simulink model "dcmotor"  (R2020b)
settings: Solver=VariableStepAuto  StartTime=0.0  StopTime=10.0  RelTol=1e-3
settings Model: Creator=Aftab  LastModifiedBy=Aftab
settings DebuggingCC: SFMachineParentedDataDiag=error

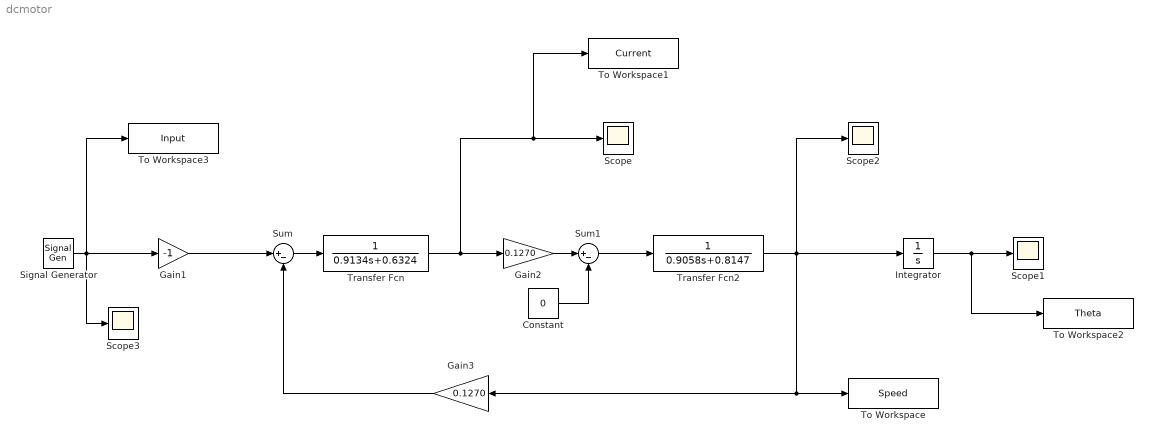
== system dcmotor ==
  Constant : Constant  Value=0
  Gain1 : Gain  Gain=-1
  Gain2 : Gain  Gain=0.1270
  Gain3 : Gain  Gain=0.1270
  Integrator : Integrator
  Scope{,1..3} (4 alike) : Scope
  Signal Generator : SignalGenerator  WaveForm=square  Amplitude=5  Frequency=1/50
  Sum : Sum  Inputs=|+-
  Sum1 : Sum  Inputs=|+-
  To Workspace : ToWorkspace  VariableName=Speed  SaveFormat=Timeseries  SampleTime=-1
  To Workspace1 : ToWorkspace  VariableName=Current  SaveFormat=Timeseries  SampleTime=-1
  To Workspace2 : ToWorkspace  VariableName=Theta  SaveFormat=Timeseries  SampleTime=-1
  To Workspace3 : ToWorkspace  VariableName=Input  SaveFormat=Timeseries  SampleTime=-1
  Transfer Fcn : TransferFcn  Denominator=[0.9134 0.6324]
  Transfer Fcn2 : TransferFcn  Denominator=[0.9058 0.8147]
  wires:
  Signal Generator/1 -> Scope3/1, To Workspace3/1, Gain1/1
  Gain1/1 -> Sum/1
  Sum/1 -> Transfer Fcn/1
  Transfer Fcn/1 -> To Workspace1/1, Scope/1, Gain2/1
  Gain2/1 -> Sum1/1
  Gain3/1 -> Sum/2
  Sum1/1 -> Transfer Fcn2/1
  Transfer Fcn2/1 -> Scope2/1, To Workspace/1, Gain3/1, Integrator/1
  Integrator/1 -> To Workspace2/1, Scope1/1
  Constant/1 -> Sum1/2
